simulink library "anchorTetherCtrl_cl"  (R2018b)
settings: Solver=VariableStepAuto  StartTime=0.0  StopTime=10.0  RelTol=1e-3
undefined symbols (not defined in the file): ctrl
libraries: filteredPIDController_ul x3
settings Model: Creator=Erin B  LastModifiedBy=Erin B

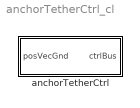
== system anchorTetherCtrl_cl ==
  anchorTetherCtrl : Subsystem

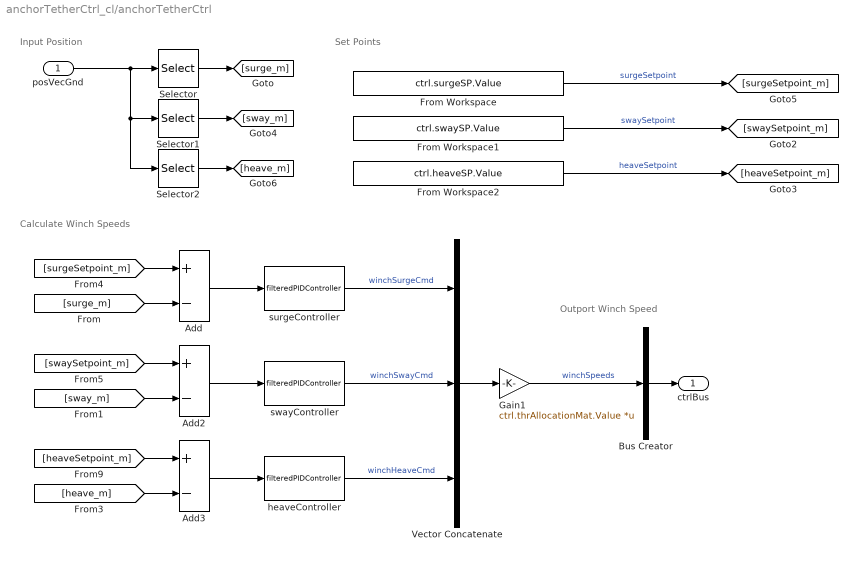
== system anchorTetherCtrl_cl/anchorTetherCtrl ==
  note: Outport Winch Speed
  note: Calculate Winch Speeds
  note: Input Position
  note: Set Points
  posVecGnd : Inport
  Add : Sum  Inputs=+-
  Add2 : Sum  Inputs=+-
  Add3 : Sum  Inputs=+-
  Bus Creator : BusCreator  Inputs=1  OutDataTypeStr=Bus: ctrlBus
  From Workspace : FromWorkspace  VariableName=ctrl.surgeSP.Value  SampleTime=0
  From Workspace1 : FromWorkspace  VariableName=ctrl.swaySP.Value  SampleTime=0
  From Workspace2 : FromWorkspace  VariableName=ctrl.heaveSP.Value  SampleTime=0
  Gain1 : Gain  Gain=ctrl.thrAllocationMat.Value  Multiplication=Matrix(K*u)
  Selector : Selector  InputPortWidth=3  IndexOptions=Index vector (dialog)  Indices=1  OutputSizes=1
  Selector1 : Selector  InputPortWidth=3  IndexOptions=Index vector (dialog)  Indices=2  OutputSizes=1
  Selector2 : Selector  InputPortWidth=3  IndexOptions=Index vector (dialog)  Indices=3  OutputSizes=1
  Vector Concatenate : Concatenate  NumInputs=3
  heaveController : filteredPIDController_ul/filteredPIDController  kp=ctrl.heave.kp.Value  ki=ctrl.heave.ki.Value  kd=ctrl.heave.kd.Value  Value=ctrl.heave.tau.Value
  surgeController : filteredPIDController_ul/filteredPIDController  kp=ctrl.surge.kp.Value  ki=ctrl.surge.ki.Value  kd=ctrl.surge.kd.Value  Value=ctrl.surge.tau.Value
  swayController : filteredPIDController_ul/filteredPIDController  kp=ctrl.sway.kp.Value  ki=ctrl.sway.ki.Value  kd=ctrl.sway.kd.Value  Value=ctrl.sway.tau.Value
  ctrlBus : Outport  OutDataTypeStr=Bus: ctrlBus
  wires:
  Add3/1 -> heaveController/1
  Add2/1 -> swayController/1
  [swaySetpoint_m] -> Add2/1
  From Workspace/1 -> [surgeSetpoint_m]  "surgeSetpoint"
  [heaveSetpoint_m] -> Add3/1
  Bus Creator/1 -> ctrlBus/1
  surgeController/1 -> Vector Concatenate/1  "winchSurgeCmd"
  Add/1 -> surgeController/1
  [sway_m] -> Add2/2
  [heave_m] -> Add3/2
  heaveController/1 -> Vector Concatenate/3  "winchHeaveCmd"
  posVecGnd/1 -> Selector1/1, Selector2/1, Selector/1
  swayController/1 -> Vector Concatenate/2  "winchSwayCmd"
  [surgeSetpoint_m] -> Add/1
  Vector Concatenate/1 -> Gain1/1
  From Workspace1/1 -> [swaySetpoint_m]  "swaySetpoint"
  From Workspace2/1 -> [heaveSetpoint_m]  "heaveSetpoint"
  Selector/1 -> [surge_m]
  Selector2/1 -> [heave_m]
  Selector1/1 -> [sway_m]
  Gain1/1 -> Bus Creator/1  "winchSpeeds"
  [surge_m] -> Add/2
